simulink model "Modulador_Analogico_UnUsuario"  (R2018b)
settings: Solver=FixedStepAuto  StartTime=0.0  StopTime=M*CantBit  FixedStep=Tsampling  RelTol=1e-3
values from neighbouring files (symbols this model uses):
  EsOFDM = 2    [Script_configParametros_Unusuario.m]
  F1 = FsepOFDM*2    [Script_configParametros_Unusuario.m]
  F2 = FsepOFDM*3    [Script_configParametros_Unusuario.m]
  F3 = FsepOFDM*4    [Script_configParametros_Unusuario.m]
  F4 = FsepOFDM*5    [Script_configParametros_Unusuario.m]
  RbOFDM = RsOFDM*sum(TransfBitPerSimb)    [Script_configParametros_Unusuario.m]
  Ts1 = Tb1    (= 0.001)    [Script_configParametros_Unusuario.m]
  Ts2 = Tb2    (= 0.001)    [Script_configParametros_Unusuario.m]
  Ts3 = Tb3    (= 0.001)    [Script_configParametros_Unusuario.m]
  Ts4 = Tb4    (= 0.001)    [Script_configParametros_Unusuario.m]
  Tsampling = M/N    [Script_configParametros_Unusuario.m]
libraries: commdigbbndpm3 x4, commrandsrc3 x1
settings Model: Creator=lukit  LastModifiedBy=lukit

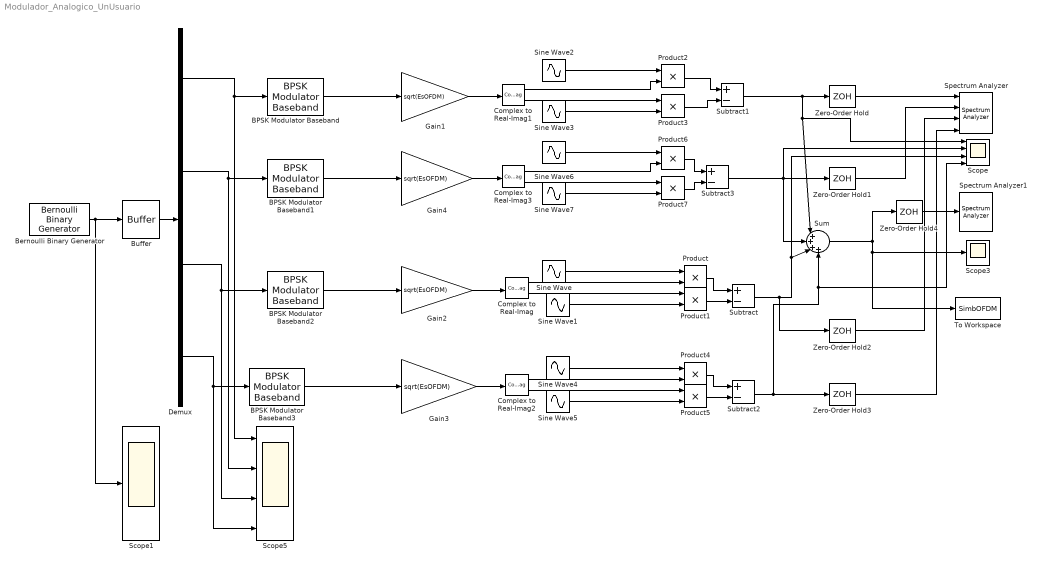
== system Modulador_Analogico_UnUsuario ==
  BPSK Modulator Baseband{,1..3} (4 alike) : commdigbbndpm3/BPSK Modulator Baseband  Ph=0  outDtype=double  outWordLen=16  outUDDataType=sfix(16)  outFracLenMode=Best precision  outFracLen=15  outDataTypeStr=double  outLastDataTypeStr=double
  Bernoulli Binary Generator : commrandsrc3/Bernoulli Binary Generator  ProbabilityOfZero=0.5  SeedSource=Auto  Seed=0  SampleTime=1/RbOFDM  SamplesPerFrame=1  OutputDataType=double  SimulateUsing=Interpreted execution
  Buffer : Buffer  N=4  OutputFrames=off
  Complex to Real-Imag{,1..3} (4 alike) : ComplexToRealImag
  Demux : Demux
  Gain{1..4} (4 alike) : Gain  Gain=sqrt(EsOFDM)
  Product{,1..7} (8 alike) : Product
  Scope : Scope  NumInputPorts=4
  Scope1 : Scope
  Scope3 : Scope
  Scope5 : Scope  NumInputPorts=4
  Sine Wave : Sin  Amplitude=sqrt(2/Ts3)  Frequency=2*pi*F3  Phase=pi/2  SampleTime=Tsampling
  Sine Wave1 : Sin  Amplitude=sqrt(2/Ts3)  Frequency=2*pi*F3  SampleTime=Tsampling
  Sine Wave2 : Sin  Amplitude=sqrt(2/Ts1)  Frequency=2*pi*F1  Phase=pi/2  SampleTime=Tsampling
  Sine Wave3 : Sin  Amplitude=sqrt(2/Ts1)  Frequency=2*pi*F1  SampleTime=Tsampling
  Sine Wave4 : Sin  Amplitude=sqrt(2/Ts4)  Frequency=2*pi*F4  Phase=pi/2  SampleTime=Tsampling
  Sine Wave5 : Sin  Amplitude=sqrt(2/Ts4)  Frequency=2*pi*F4  SampleTime=Tsampling
  Sine Wave6 : Sin  Amplitude=sqrt(2/Ts2)  Frequency=2*pi*F2  Phase=pi/2  SampleTime=Tsampling
  Sine Wave7 : Sin  Amplitude=sqrt(2/Ts2)  Frequency=2*pi*F2  SampleTime=Tsampling
  Spectrum Analyzer : SpectrumAnalyzer  NumInputPorts=4
  Spectrum Analyzer1 : SpectrumAnalyzer
  Subtract{,1..3} (4 alike) : Sum  Inputs=+-
  Sum : Sum  Inputs=|++++
  To Workspace : ToWorkspace  VariableName=SimbOFDM  SampleTime=Tsampling
      settings: Save2DSignal=2-D array (concatenate along first dimension)
  Zero-Order Hold{,1..4} (5 alike) : ZeroOrderHold  SampleTime=-1
  wires:
  Product/1 -> Subtract/1
  Product1/1 -> Subtract/2
  Sine Wave/1 -> Product/1
  Sine Wave1/1 -> Product1/2
  Complex to Real-Imag/2 -> Product1/1
  Complex to Real-Imag/1 -> Product/2
  Gain2/1 -> Complex to Real-Imag/1
  Sine Wave2/1 -> Product2/1
  Complex to Real-Imag1/1 -> Product2/2
  Sine Wave3/1 -> Product3/2
  Complex to Real-Imag1/2 -> Product3/1
  Gain1/1 -> Complex to Real-Imag1/1
  Product2/1 -> Subtract1/1
  Product3/1 -> Subtract1/2
  BPSK Modulator Baseband/1 -> Gain1/1
  Subtract/1 -> Zero-Order Hold2/1, Scope/3, Sum/3
  Product4/1 -> Subtract2/1
  Sine Wave4/1 -> Product4/1
  Product5/1 -> Subtract2/2
  Sine Wave5/1 -> Product5/2
  Subtract2/1 -> Zero-Order Hold3/1, Scope/4, Sum/4
  Complex to Real-Imag2/2 -> Product5/1
  Gain3/1 -> Complex to Real-Imag2/1
  BPSK Modulator Baseband1/1 -> Gain4/1
  Sine Wave6/1 -> Product6/1
  Complex to Real-Imag3/1 -> Product6/2
  Sine Wave7/1 -> Product7/2
  Product6/1 -> Subtract3/1
  Product7/1 -> Subtract3/2
  Complex to Real-Imag3/2 -> Product7/1
  Gain4/1 -> Complex to Real-Imag3/1
  Sum/1 -> To Workspace/1, Scope3/1, Zero-Order Hold4/1
  Zero-Order Hold/1 -> Spectrum Analyzer/1
  Zero-Order Hold1/1 -> Spectrum Analyzer/2
  Zero-Order Hold2/1 -> Spectrum Analyzer/3
  Zero-Order Hold3/1 -> Spectrum Analyzer/4
  Zero-Order Hold4/1 -> Spectrum Analyzer1/1
  BPSK Modulator Baseband3/1 -> Gain3/1
  BPSK Modulator Baseband2/1 -> Gain2/1
  Subtract3/1 -> Zero-Order Hold1/1, Sum/2, Scope/2
  Subtract1/1 -> Sum/1, Scope/1, Zero-Order Hold/1
  Buffer/1 -> Demux/1
  Bernoulli Binary Generator/1 -> Scope1/1, Buffer/1
  Demux/1 -> BPSK Modulator Baseband/1, Scope5/1
  Demux/2 -> BPSK Modulator Baseband1/1, Scope5/2
  Demux/3 -> BPSK Modulator Baseband2/1, Scope5/3
  Demux/4 -> BPSK Modulator Baseband3/1, Scope5/4
  Complex to Real-Imag2/1 -> Product4/2
